simulink model "LiepkePlane"  (R2021a)
settings: Solver=FixedStepDiscrete  StartTime=0.0  StopTime=100  RelTol=1e-3  EnableMultiTasking=on
InitFcn:
  | runStart
StopFcn:
  | createGraphs
values from neighbouring files (symbols this model uses):
  alpha_matrix = data.alpha    [DatcomImport.m]
  alphai = trimAngle    (= -0.08927272)    [runStart.m]
  alt_matrix = data.alt    [DatcomImport.m]
  b = 8.0162    [runStart.m]
  beta = 0    [runStart.m]
  cbar = 4.3    [runStart.m]
  CD_0 = 0.0205    [runStart.m]
  CD_alpha = 0.058388    [runStart.m]
  CD_de = 0    [runStart.m]
  CD_ih = 0    [runStart.m]
  CD_q = 0    [runStart.m]
  CL_0 = 0.149    [runStart.m]
  Cl_0 = 0    [runStart.m]
  CL_alpha = 5.1265    [runStart.m]
  Cl_beta = -0.0301    [runStart.m]
  Cl_da = -0.1    [runStart.m]
  CL_de = 0.38    [runStart.m]
  Cl_dr = 0.05    [runStart.m]
  CL_ih = 0    [runStart.m]
  Cl_p = -0.5    [runStart.m]
  CL_q = 10.0    (= 10)    [runStart.m]
  Cl_r = 0.28    [runStart.m]
  cla_matrix = data.cla    [DatcomImport.m]
  clb_matrix = data.clb    [DatcomImport.m]
  clp_matrix = data.clp    [DatcomImport.m]
  clq_matrix = data.clq    [DatcomImport.m]
  clr_matrix = data.clr    [DatcomImport.m]
  Cm_0 = -0.08    [runStart.m]
  Cm_alpha = -0.3109    [runStart.m]
  Cm_de = -0.88    [runStart.m]
  Cm_ih = 0    [runStart.m]
  Cm_q = -17.7    [runStart.m]
  cma_matrix = data.cma    [DatcomImport.m]
  cmq_matrix = data.cmq    [DatcomImport.m]
  Cn_0 = 0    [runStart.m]
  Cn_beta = 0.1297    [runStart.m]
  Cn_da = 0.003    [runStart.m]
  Cn_dr = -0.18436    [runStart.m]
  Cn_p = - 0.09    (= -0.09)    [runStart.m]
  Cn_r = -0.26    [runStart.m]
  cnb_matrix = data.cnb    [DatcomImport.m]
  cnp_matrix = data.cnp    [DatcomImport.m]
  cnr_matrix = data.cnr    [DatcomImport.m]
  CY_0 = 0    [runStart.m]
  CY_beta = -.0301    (= -0.0301)    [runStart.m]
  CY_da = 0    [runStart.m]
  CY_dr = 0.0280    (= 0.028)    [runStart.m]
  CY_p = -0.140    (= -0.14)    [runStart.m]
  CY_r = 0.61    [runStart.m]
  cyb_matrix = data.cyb    [DatcomImport.m]
  cyp_matrix = data.cyp    [DatcomImport.m]
  H = 1981.2    [runStart.m]
  Ix = 1084.7    [runStart.m]
  Iy = 6507.9    [runStart.m]
  Iz = 7050.3    [runStart.m]
  Jxy = 0    [runStart.m]
  Jxz = 271.16    [runStart.m]
  Jyz = 0    [runStart.m]
  m = 2267.9    [runStart.m]
  mach_matrix = data.mach    [DatcomImport.m]
  p = 0    [runStart.m]
  phi = 0    [runStart.m]
  psi = 0    [runStart.m]
  q = 0    [runStart.m]
  r = 0    [runStart.m]
  S = 12.6348    [runStart.m]
  theta = trimAngle    (= -0.08927272)    [runStart.m]
  trimAngle = -8.927272e-02    (= -0.08927272)    [runStart.m]
  trimThrotte = 3.827652e-01    (= 0.3827652)    [runStart.m]
  v = 180    [runStart.m]
  xe = 0    [runStart.m]
  ye = 0    [runStart.m]
undefined symbols (not defined in the file or in its folder): DiscIntNeverNeededParam
libraries: airlib x2, aerolibfltsims x2, aerolibanimutils x2
(part 1 of 2)
settings Model: Creator=MONCAYOH  LastModifiedBy=matt
settings SolverCC: AlgebraicLoopSolver=TrustRegion
settings DataIOCC: SaveFormat=Array  SignalLoggingSaveFormat=ModelDataLogs  SaveOutput=off  SaveTime=off  ReturnWorkspaceOutputs=off
settings OptimizationCC: BlockReduction=off  BooleanDataType=off
settings DebuggingCC: SaveWithParameterizedLinksMsg=none  UnderspecifiedInitializationDetection=Classic  MergeDetectMultiDrivingBlocksExec=none  SignalResolutionControl=TryResolveAllWithWarning  MultiTaskDSMMsg=warning  MultiTaskCondExecSysMsg=none  SFMachineParentedDataDiag=warning  ArithmeticOperatorsInVariantConditions=warning
settings HardwareCC: TargetUnknown=on
settings ModelReferenceCC: PropagateSignalLabelsOutOfModel=off
settings SFSimCC: SimUseLocalCustomCode=off  CustomCodeUndefinedFunction=UseInterfaceOnly
settings RTWCC: RTWUseLocalCustomCode=off
settings CodeAppCC: StateflowObjectComments=on
settings GRTTargetCC: TargetLangStandard=C89/C90 (ANSI)  CombineOutputUpdateFcns=off  GRTInterface=on

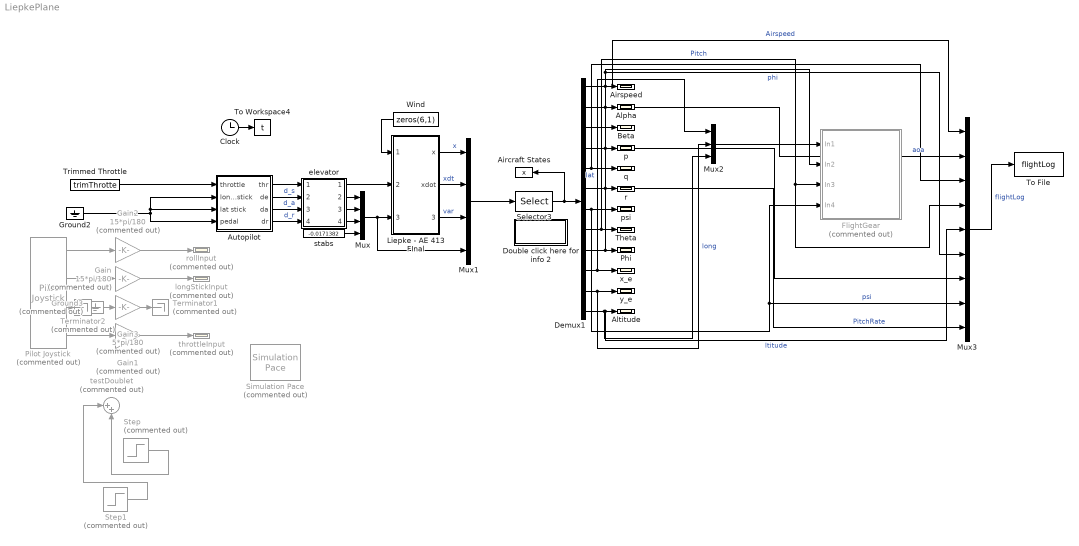
== system LiepkePlane ==
  " Liepke - AE 413 FInal" : Subsystem  AncestorBlock=airlib/B747  mask(General Nonlinear Aircraft Model){GM1=[cbar   b   S   Ix  Iy  Iz   Jxy Jxz  Jyz   m], CD_wind=[CD_0   CD_alpha   CD_q   CD_de   CD_ih], CL_wind=[CL_0   CL_alpha   CL_q   CL_de   CL_ih], Cm_body=[Cm_0   Cm_alpha   Cm_q   Cm_de   Cm_ih], CY_body=[CY_0   CY_beta   CY_p   CY_r   CY_da   CY_dr], Cl_body=[Cl_0   Cl_beta   Cl_p   Cl_r   Cl_da   Cl_dr], Cn_body=[Cn_0   Cn_beta   Cn_p   Cn_r   Cn_da   Cn_dr], x0=[v alphai beta p q r psi theta phi xe ye H]}
      mask prompts: GM1 "Geometry and Mass : [cbar   b    S    Ix   Iy   Iz   Jxy  Jxz  Jyz  m]"; CD_wind "Aerodynamic D-Force Derivatives : [CD0 CDa CDq CDde CDih]"; CL_wind "Aerodynamic L-Force Derivatives : [CL0 CLa CLq CLde CLih]"; Cm_body "Aerodynamic Y-Moment Derivatives : [Cm0 Cma Cmq Cmde Cmih]"; CY_body "Aerodynamic Y-Force Derivatives : [CY0 CYb CYp CYr CYda CYdr]"; Cl_body "Aerodynamic X-moment Derivatives : [Cl0 Clb Clp Clr Clda Cldr]"; Cn_body "Aerodynamic Z-moment Derivatives : [Cn0 Cnb Cnp Cnr Cnda Cndr]"; x0 "Initial Condition x0 [v alpha beta p q r psi theta phi xe ye H]"
      mask help:
      | The first input contains the wind velocity and acceleration.
      |   The second input contains external forces and moments in body axis.
      |   The third input contains the deflections of elevators, ailerons, rudder,
      |   and flaps. For a list of outputs look under the mask.
      |   NB : The International measurement system (MKS) is adopted.
      mask init:
      | AM=zeros(6,19);
      | AM(1,[1 2 9 11 12])=reshape(CD_wind,1,5);
      | AM(3,[1 2 9 11 12])=reshape(CL_wind,1,5);
      | AM(5,[1 2 9 11 12])=reshape(Cm_body,1,5);
      | AM(2,[1 5 8 10 13 14])=reshape(CY_body,1,6);
      | AM(4,[1 5 8 10 13 14])=reshape(Cl_body,1,6);
      | AM(6,[1 5 8 10 13 14])=reshape(Cn_body,1,6);
      | 
      | Ix=GM1(4);Iy=GM1(5);Iz=GM1(6);
      | Jxy=GM1(7);Jxz=GM1(8);Jyz=GM1(9);
      | 
      | detI = Ix*Iy*Iz - 2*Jxy*Jxz*Jyz - Ix*Jyz^2 - Iy*Jxz^2 - Iz*Jxy^2;
      | I1   = Iy*Iz - Jyz^2;I2   = Jxy*Iz + Jyz*Jxz;
      | I3   = Jxy*Jyz + Iy*Jxz;I4   = Ix*Iz - Jxz^2;
      | I5   = Ix*Jyz + Jxy*Jxz;I6   = Ix*Iy - Jxy^2;
      | 
      | Pl  = I1/detI; Pm = I2/detI; Pn = I3/detI;
      | Ppp = -(Jxz*I2 - Jxy*I3)/detI;Ppq = (Jxz*I1 - Jyz*I2 - (Iy-Ix)*I3)/detI;
      | Ppr = -(Jxy*I1 + (Ix-Iz)*I2 - Jyz*I3)/detI;Pqq = (Jyz*I1 - Jxy*I3)/detI;
      | Pqr = -((Iz-Iy)*I1 - Jxy*I2 + Jxz*I3)/detI;Prr = -(Jyz*I1 - Jxz*I2)/detI;
      | 
      | Ql  = I2/detI; Qm = I4/detI; Qn = I5/detI;
      | Qpp = -(Jxz*I4 - Jxy*I5)/detI;Qpq = (Jxz*I2 - Jyz*I4 - (Iy-Ix)*I5)/detI;
      | Qpr = -(Jxy*I2 + (Ix-Iz)*I4 - Jyz*I5)/detI;Qqq = (Jyz*I2 - Jxy*I5)/detI;
      | Qqr = -((Iz-Iy)*I2 - Jxy*I4 + Jxz*I5)/detI;Qrr = -(Jyz*I2 - Jxz*I4)/detI;
      | 
      | Rl  = I3/detI; Rm = I5/detI; Rn = I6/detI;
      | Rpp = -(Jxz*I5 - Jxy*I6)/detI;
      | Rpq = (Jxz*I3 - Jyz*I5 - (Iy-Ix)*I6)/detI;
      | Rpr = -(Jxy*I3 + (Ix-Iz)*I5 - Jyz*I6)/detI;
      | Rqq = (Jyz*I3 - Jxy*I6)/detI;
      | Rqr = -((Iz-Iy)*I3 - Jxy*I5 + Jxz*I6)/detI;
      | Rrr = -(Jyz*I3 - Jxz*I5)/detI;
      | 
      | GM2 = [  Pl   Pm   Pn   Ppp  Ppq  Ppr  Pqq  Pqr  Prr ;
      |                Ql  Qm   Qn   Qpp  Qpq  Qpr  Qqq  Qqr  Qrr ;
      |                Rl  Rm   Rn   Rpp  Rpq  Rpr  Rqq  Rqr  Rrr ];
      | 
      | xfix=1;
      mask Help:
      | <p>
      | This block is a general nonlinear 6DOF aircraft model, with a very accurate built-in atmosphere model and constant aerodynamic derivatives.
      | The architecture of the block is largely based on the Aircraft block provided by the <A
      | HREF="http://www.mathworks.com/matlabcentral/fileexchange/loadFile.do?objectId=252&objectType=file">FDC toolbox</A> (Marc Rauw, 1993-2000).
      | </p>
      | <p>
      | The geometric and inertal data of the aircraft are entered as parameters in the first row of the mask. The other six rows contains the
      | non-dimensional aerodynamic derivatives. The last row is the initial state.
      | </p>
      | <p>
      | The first input contains the wind velocity and acceleration.
      | The second input contains external forces and moments in the aircraft body axis.
      | The third input contains the deflections of elevators, ailerons, rudder,
      | and flaps or stabilators. For a list of outputs look under the mask.
      | </p>
      | <p>
      | The control surface sign conventions are the same adopted in books such as Stevens-Lewis and Etkin, and in many flight simulators,
      | including the FDC toolbox. <br>
      | Specifically, positive elevator deflection causes negative pitching moment (Cmde &#60 0), positive rudder deflection causes negative yawing
      | moment (Cndr &#60 0), and positive aileron deflection causes negative rolling moment (Clda &#60 0). Another way to say the same thing is
      | that, the positive elevators deflection is Trailing Edge Down (TED), the positive rudder(s) deflection is Trailing Edge Left (TEL), and,
      | taking as TED the positive ailerons deflection, da=K*(da_right-da_left), with K usually equal to 1 (FDC) or 1/2.
      | </p>
      | <p>
      | Since this block is largely based on the FDC toolbox, i redirect you to the FDC Toolbox manual, for a good explanation of the underlying
      | components. Besides the mask and the fact that the aerodynamic derivatives are expressed in the stability axis, the only relevant difference
      | with the FDC toolbox is that in the computation of the aerodynamic forces, q is normalized as q*cbar/2V instead of q*cbar/V. The majority
      | of aeronautics books that i've seen use q*cbar/2V.
      | </p>
      | <p>
      | Please note that the International Measurement System is adopted. So, lengths are in meters, masses in Kg, and inertia moments in Kg*m^2.
      | Moreover, forces are in N, moments in N*m, accelerations in g, and angles in radians. For those that use the english system, here are some useful
      | conversion factors: <br>
      | 1 ft   = 0.3048 m, 1 lb   = 0.4536 Kg, 1 slug = 14.593903 Kg ,  1 slug*ft^2 = 1.355818 Kg*m^2
      | <br>
      | </p>
      | <p>
      | Finally, there is an <A HREF="http://www.aae.uiuc.edu/m-selig/apasim/Aircraft-uiuc.html">excellent source</A> of aircraft aerodynamic data
      | which is mantained by Michael S. Selig, Rob Deters, and Glen Dimock at the university of Urbana-Champaign. To use any of the given models
      | you just need to type the supplied aircraft data in the block mask.
      | </p>
      | <p>
      | <p>
      | December 2002, Giampiero Campa
      | </p>
      | </p>
      mask Display: disp('General\nAircraft\nModel')
  Aircraft States : ToWorkspace  VariableName=x  SampleTime=0.05
  Airspeed : Scope
  Alpha : Scope
  Altitude : Scope
  Autopilot : Subsystem
  Beta : Scope
  Clock : Clock
  Demux1 : Demux  Outputs=12
      settings: DisplayOption=none
  Double click here for info 2 : Subsystem
      mask Display: disp('Output\nSignals')
  FlightGear : Subsystem  Commented=on
  Gain : Gain  Commented=on  Gain=15*pi/180
  Gain1 : Gain  Commented=on
  Gain2 : Gain  Commented=on  Gain=15*pi/180
  Gain3 : Gain  Commented=on  Gain=5*pi/180
  Ground2 : Ground
  Ground3 : Ground  Commented=on
  Mux : Mux
  Mux1 : Mux  Inputs=[12 12 12 4]
  Mux2 : Mux  Inputs=3
  Mux3 : Mux  Inputs=9
  Phi : Scope
  Pilot Joystick : aerolibanimutils/Pilot Joystick  Commented=on  JoystickID=Joystick1  OutputConfiguration=FourAxis  SampleTime=.05
  Selector3 : Selector  InputPortWidth=40  IndexOptions=Index vector (dialog)  Indices=1:12  OutputSizes=1
  Simulation Pace : aerolibanimutils/Simulation Pace  Commented=on  SimulationPace=1  SleepMode=Auto  OutputPaceError=off  SampleTime=-1
  Step : Step  Commented=on  Time=2  Before=-1  SampleTime=0
  Step1 : Step  Commented=on  Time=4  After=-1  SampleTime=0
  Terminator1 : Terminator  Commented=on
  Terminator2 : Terminator  Commented=on
  Theta : Scope
  To File : ToFile  Filename=flightLog  MatrixName=data  SaveFormat=Timeseries
  To Workspace4 : ToWorkspace  VariableName=t  SampleTime=-1
  Trimmed Throttle : Constant  Value=trimThrotte
  Wind : Constant  Value=zeros(6,1)
  elevator : Subsystem
      mask Display: disp('Cable &\nactuator\ndynamics')
  longStickInput : Scope  Commented=on
  p : Scope
  psi : Scope
  q : Scope
  r : Scope
  rollInput : Scope  Commented=on
  stabs : Constant  Value=-0.0171382
  testDoublet : Sum  Commented=on  Inputs=|++
  throttleInput : Scope  Commented=on
  x_e : Scope
  y_e : Scope
  wires:
  elevator/3(deltaa) -> Mux/2
  elevator/4(deltar) -> Mux/3
  elevator/2(deltae) -> Mux/1
  Autopilot/2(de) -> elevator/2(D_elv)  "d_s"
  Autopilot/3(da) -> elevator/3(D_ail)  "d_a"
  Autopilot/4(dr) -> elevator/4(D_rud)  "d_r"
  Mux/1 -> " Liepke - AE 413 FInal"/3(deflect), Mux1/4
  elevator/1(throttle) -> " Liepke - AE 413 FInal"/2(ext fm)
  Selector3/1 -> Demux1/1, Aircraft States/1
  Demux1/3 -> Beta/1
  Demux1/4 -> Mux3/7, p/1
  Demux1/5 -> q/1, Mux3/3
  Demux1/7 -> Mux3/8, FlightGear/4(In4), psi/1  "psi"
  Demux1/9 -> Mux3/6, FlightGear/2(In2), Phi/1  "phi"
  Demux1/10 -> Mux2/1, x_e/1  "lat"
  Demux1/11 -> Mux2/2, y_e/1  "long"
  Autopilot/1(thr) -> elevator/1(D_thr)
  Clock/1 -> To Workspace4/1
  stabs/1 -> Mux/4
  Wind/1 -> " Liepke - AE 413 FInal"/1(" uwind")
  " Liepke - AE 413 FInal"/1(x) -> Mux1/1  "x"
  " Liepke - AE 413 FInal"/2(xdot) -> Mux1/2  "xdt"
  " Liepke - AE 413 FInal"/3(others) -> Mux1/3  "var"
  Mux2/1 -> FlightGear/1(In1)
  Mux1/1 -> Selector3/1
  Demux1/12 -> Mux3/5, Altitude/1, Mux2/3  "ltitude"
  Demux1/2 -> Mux3/2, Alpha/1  "aoa"
  Demux1/8 -> Mux3/4, FlightGear/3(In3), Theta/1  "Pitch"
  Demux1/1 -> Mux3/1, Airspeed/1  "Airspeed"
  Mux3/1 -> To File/1  "flightLog"
  Demux1/6 -> Mux3/9, r/1  "PitchRate"
  Gain1/1 -> throttleInput/1
  Pilot Joystick/3 -> Terminator2/1
  Step1/1 -> testDoublet/1
  Step/1 -> testDoublet/2
  Gain2/1 -> rollInput/1
  Gain/1 -> longStickInput/1
  Pilot Joystick/1 -> Gain2/1
  Pilot Joystick/2 -> Gain/1
  Pilot Joystick/4 -> Gain1/1
  Ground2/1 -> Autopilot/3(lat stick), Autopilot/2(long stick), Autopilot/4(pedal)
  Trimmed Throttle/1 -> Autopilot/1(throttle)
  Gain3/1 -> Terminator1/1
  Ground3/1 -> Gain3/1

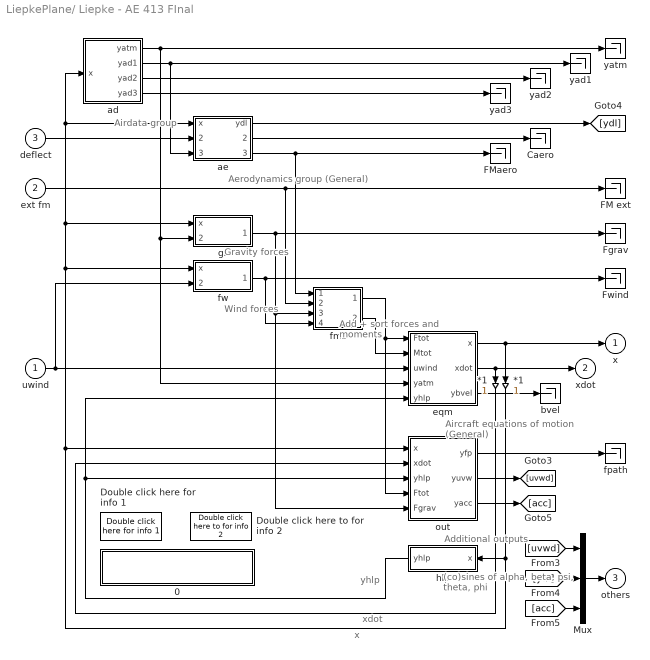
== system LiepkePlane/ Liepke - AE 413 FInal ==
  note: xdot
  note: x
  note: yhlp
  note: Additional outputs
  note: Aircraft equations
      | of motion (General)
  note: Wind forces
  note: Gravity forces
  note: Aerodynamics
      | group (General)
  note: (co)sines of
      | alpha, beta,
      | psi, theta, phi
  note: Add + sort
      | forces and
      | moments
  note: Airdata group
  " uwind" : Inport
  ext fm : Inport  Port=2
  deflect : Inport  Port=3
  " *1" : Gain  SaturateOnIntegerOverflow=on  OutDataTypeStr=Inherit: Same as input  ParamDataTypeStr=Inherit: Same as input
  *1 : Gain  SaturateOnIntegerOverflow=on  OutDataTypeStr=Inherit: Same as input  ParamDataTypeStr=Inherit: Same as input
  0 : Subsystem
      mask Display: disp('AIRCRAFT, main level\nM.O. Rauw')
  Caero : Terminator
  Double click here for info 1 : airlib/DT-B747/Double click here for info 1  SystemSampleTime=-1  VariantActivationTime=update diagram  Latency=0  AutoFrameSizeCalculation=off
  Double click here to for info 2 : airlib/DT-B747/Double click here to for info 2  SystemSampleTime=-1  VariantActivationTime=update diagram  Latency=0  AutoFrameSizeCalculation=off
  FM ext : Terminator
  FMaero : Terminator
  Fgrav : Terminator
  Fwind : Terminator
  Mux : Mux  Inputs=[3 3 6]
  ad : Subsystem
  ae : Subsystem
  bvel : Terminator
  eqm : Subsystem
  fms : Subsystem  mask(FMsort){}
      mask help: Forces and Moments sorting block
      mask Display: disp('FMsort')
  fpath : Terminator
  fw : Subsystem  mask(fwind){m=GM1(10)}
      mask prompts: m "Mass of the aircraft [kg]:"
      mask help: Forces due to non-steady atmosphere.
      mask Display: disp('Fwind')
  gr : Subsystem  mask(Gravity){m=GM1(10)}
      mask prompts: m "Mass of the aircraft [kg]:"
      mask help: Gravity forces.
      mask Display: disp('Gravity')
  hlp : Subsystem  mask(Hlpfcn){}
      mask help: Help sines and cosines
      mask Display: disp('hlpfcn')
  out : Subsystem
  yad1 : Terminator
  yad2 : Terminator
  yad3 : Terminator
  yatm : Terminator
  x : Outport
  xdot : Outport  Port=2
  others : Outport  Port=3
  wires:
  fms/1(Ftot) -> out/4(Ftot), eqm/1(Ftot)
  ext fm/1 -> fms/2(FMprop), FM ext/1
  deflect/1 -> ae/2(uaero)
  ad/4(yad3) -> yad3/1
  ae/1(ydl) -> [ydl]
  ae/2(Caero) -> Caero/1
  eqm/3(ybvel) -> bvel/1
  out/1(yfp) -> fpath/1
  ad/2(yad1) -> ae/3(yad1), yad1/1
  ad/3(yad2) -> yad2/1
  ad/1(yatm) -> eqm/4(yatm), gr/2(yatm), yatm/1
  out/3(yacc) -> [acc]
  fw/1(Fwind) -> Fwind/1, fms/4(Fwind)
  ae/3(FMaero) -> FMaero/1, fms/1(FMaero)
  hlp/1(yhlp) -> eqm/5(yhlp), out/3(yhlp)
  " uwind"/1 -> eqm/3(uwind), fw/2(uwind)
  *1/1 -> out/2(xdot)
  gr/1(Fgrav) -> fms/3(Fgrav), out/5(Fgrav), Fgrav/1
  " *1"/1 -> hlp/1(x), out/1(x), fw/1(x), gr/1(x), ae/1(x), ad/1(x)
  eqm/2(xdot) -> xdot/1, *1/1
  eqm/1(x) -> x/1, " *1"/1
  fms/2(Mtot) -> eqm/2(Mtot)
  out/2(yuvw) -> [uvwd]
  [uvwd] -> Mux/1
  [ydl] -> Mux/2
  [acc] -> Mux/3
  Mux/1 -> others/1

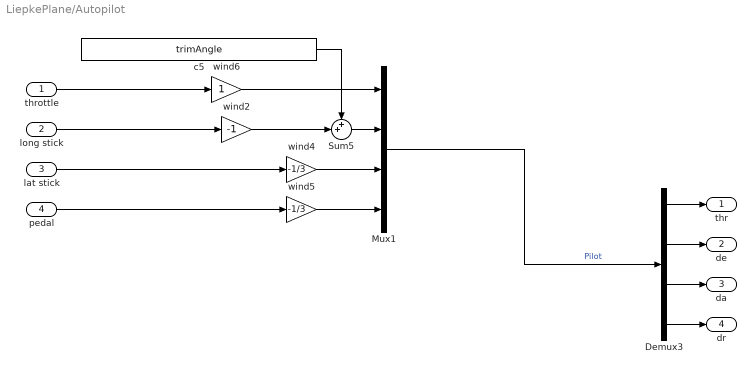
== system LiepkePlane/Autopilot ==
  throttle : Inport
  long stick : Inport  Port=2
  lat stick : Inport  Port=3
  pedal : Inport  Port=4
  Demux3 : Demux
      settings: DisplayOption=none
  Mux1 : Mux
  Sum5 : Sum  Inputs=++|  InputSameDT=on  SaturateOnIntegerOverflow=on  OutDataTypeStr=Inherit: Same as first input
  c5 : Constant  Value=trimAngle
  wind2 : Gain  Gain=-1  SaturateOnIntegerOverflow=on  OutDataTypeStr=Inherit: Same as input  ParamDataTypeStr=Inherit: Same as input
  wind4 : Gain  Gain=-1/3  SaturateOnIntegerOverflow=on  OutDataTypeStr=Inherit: Same as input  ParamDataTypeStr=Inherit: Same as input
  wind5 : Gain  Gain=-1/3  SaturateOnIntegerOverflow=on  OutDataTypeStr=Inherit: Same as input  ParamDataTypeStr=Inherit: Same as input
  wind6 : Gain  SaturateOnIntegerOverflow=on  OutDataTypeStr=Inherit: Same as input  ParamDataTypeStr=Inherit: Same as input
  thr : Outport  VectorParamsAs1DForOutWhenUnconnected=off
  de : Outport  Port=2  VectorParamsAs1DForOutWhenUnconnected=off
  da : Outport  Port=3  VectorParamsAs1DForOutWhenUnconnected=off
  dr : Outport  Port=4  VectorParamsAs1DForOutWhenUnconnected=off
  wires:
  long stick/1 -> wind2/1
  lat stick/1 -> wind4/1
  pedal/1 -> wind5/1
  Mux1/1 -> Demux3/1  "Pilot"
  Demux3/1 -> thr/1
  Demux3/2 -> de/1
  Demux3/3 -> da/1
  Demux3/4 -> dr/1
  wind4/1 -> Mux1/3
  wind5/1 -> Mux1/4
  throttle/1 -> wind6/1
  c5/1 -> Sum5/1
  Sum5/1 -> Mux1/2
  wind2/1 -> Sum5/2
  wind6/1 -> Mux1/1

== system LiepkePlane/Double click here for info 2 ==
  note: 01 v (m/s)
      | 02 alpha (rad)
      | 03 beta (rad)
      | 04 p (rad/s)
      | 05 q (rad/s)
      | 06 r  (rad/s)
      | 07 psi (rad)
      | 08 theta (rad)
      | 09 phi (rad)
      | 10 xe (m)
      | 11 ye (m)
      | 12 ze (m)
      | 13 v dot (m/s2)
      | 14 alpha dot (rad/s)
      | 15 beta dot (rad/s)
      | 16 p dot (rad/s2)
      | 17 q dot (rad/s2)
      | 18 r dot (rad/s2)
      | 19 fi dot (rad/s)
      | 20 theta dot (rad/s)
      | 21 psi dot (rad/s)
      | 22 xe dot (m/s)
      | 23 ye dot (m/s)
      | 24 ze dot (m/s)
      | 25 u dot (m/s2)
      | 26 v dot (m/s2)
      | 27 w dot (m/s2)
      | 28 pb/2v (rad)
      | 29 qc/v (rad)
      | 30 rb/v (rad)
      | 31 Ax (g)
      | 32 Ay (g)
      | 33 Az (g)
      | 34 ax (g)
      | 35 ay (g)
      | 36 az (g)
      | 37 delta elevators (rad)
      | 38 delta ailerons (rad)
      | 39 delta rudder (rad)
      | 40 delta stabs (rad)

== system LiepkePlane/FlightGear ==
  In1 : Inport
  In2 : Inport  Port=2
  In3 : Inport  Port=3
  In4 : Inport  Port=4
  Data Type Conversion : DataTypeConversion  OutDataTypeStr=single
  Data Type Conversion1 : DataTypeConversion  OutDataTypeStr=single
  Data Type Conversion2 : DataTypeConversion  OutDataTypeStr=single
  Lat,Lon,Elev Convertor : Subsystem
  Pack net_fdm Packet for FlightGear : aerolibfltsims/Pack net_fdm Packet for FlightGear  FlightGearVersion=v2.4  ShowPositionAttitudeInputs=on  ShowVelocityAccelerationInputs=off  ShowControlSurfacePositionInputs=off  ShowEngineFuelInputs=off  ShowLandingGearInputs=off  ShowEnvironmentInputs=off  SampleTime=-1  packetVersion=24
      settings: SourceProductBaseCode=AE
  Send net_fdm Packet to FlightGear : aerolibfltsims/Send net_fdm Packet to FlightGear  DestinationIpAddress=127.0.0.1  DestinationPort=5502  LocalIpPort=-1  varLen=off  SampleTime=-1
      settings: SourceProductBaseCode=AE
  wires:
  In2/1 -> Data Type Conversion2/1
  In3/1 -> Data Type Conversion1/1
  Lat,Lon,Elev Convertor/2(Lat) -> Pack net_fdm Packet for FlightGear/2
  Lat,Lon,Elev Convertor/3(Ele) -> Pack net_fdm Packet for FlightGear/3
  In1/1 -> Lat,Lon,Elev Convertor/1(Inp)
  Data Type Conversion1/1 -> Pack net_fdm Packet for FlightGear/5
  Data Type Conversion2/1 -> Pack net_fdm Packet for FlightGear/4
  Lat,Lon,Elev Convertor/1(Lon) -> Pack net_fdm Packet for FlightGear/1
  In4/1 -> Data Type Conversion/1
  Data Type Conversion/1 -> Pack net_fdm Packet for FlightGear/6
  Pack net_fdm Packet for FlightGear/1 -> Send net_fdm Packet to FlightGear/1

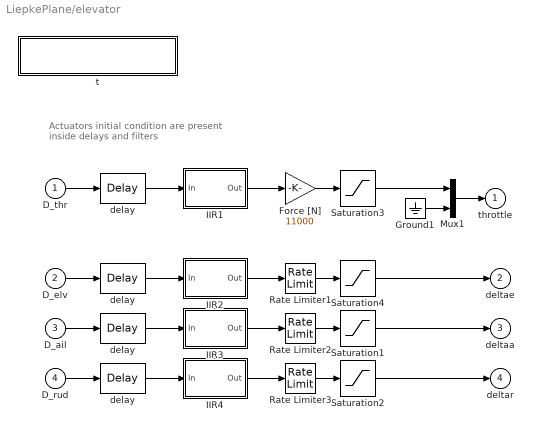
== system LiepkePlane/elevator ==
  note: Actuators initial condition are present
      | inside delays and filters
  D_thr : Inport
  D_elv : Inport  Port=2
  D_ail : Inport  Port=3
  D_rud : Inport  Port=4
  " delay" : TransportDelay  DelayTime=0.03  InitialOutput=-1.71374e-004
  " delay " : TransportDelay  DelayTime=0.03  InitialOutput=0.490154
  Force [N] : Gain  Gain=11000  SaturateOnIntegerOverflow=on  OutDataTypeStr=Inherit: Same as input  ParamDataTypeStr=Inherit: Same as input
  Ground1 : Ground
  IIR1 : Subsystem  mask(Discrete Time First Order IIR){ni=1, a=4, x0=0.490154, T=0.05}
      mask prompts: ni "Number of Channels"; a "Cutoff Frequency (a)"; x0 "Initial Condition"; T "Sample Time"
      mask help:
      | Each channel has the transfer function
      |   (1-exp(-aT))/(1-exp(-aT)(z^-1)) which is a good
      |   (pz-matched) approximation of a/(s+a) if 10*a*T<pi
      mask init:
      | A=[];B=[];C=[];D=[];
      | for i=1:ni,
      | A=[A,zeros(size(A,1),1);zeros(1,size(A,2)),exp(-a*T)];
      | B=[B,zeros(size(B,1),1);zeros(1,size(B,2)),1-exp(-a*T)];
      | C=[C,zeros(size(C,1),1);zeros(1,size(C,2)),exp(-a*T)];
      | D=[D,zeros(size(D,1),1);zeros(1,size(D,2)),1-exp(-a*T)];
      | end
      mask Help:
      | <p>
      |   Each channel has the transfer function
      |   (1-exp(-aT))/(1-exp(-aT)(z^-1)) which is a good
      |   (pz-matched) approximation of a/(s+a) if 10*a*T<pi
      | </p>
      mask Display: dpoly(a,[1 a],'s')
  IIR2 : Subsystem  mask(Discrete Time First Order IIR){ni=1, a=15, x0=-1.71374e-004, T=0.05}
      mask prompts: ni "Number of Channels"; a "Cutoff Frequency (a)"; x0 "Initial Condition"; T "Sample Time"
      mask help:
      | Each channel has the transfer function
      |   (1-exp(-aT))/(1-exp(-aT)(z^-1)) which is a good
      |   (pz-matched) approximation of a/(s+a) if 10*a*T<pi
      mask init: same as LiepkePlane/elevator/IIR1
      mask Help:
      | <p>
      |   Each channel has the transfer function
      |   (1-exp(-aT))/(1-exp(-aT)(z^-1)) which is a good
      |   (pz-matched) approximation of a/(s+a) if 10*a*T<pi
      | </p>
      mask Display: dpoly(a,[1 a],'s')
  IIR3 : Subsystem  mask(Discrete Time First Order IIR){ni=1, a=40, x0=0, T=0.05}
      mask prompts: ni "Number of Channels"; a "Cutoff Frequency (a)"; x0 "Initial Condition"; T "Sample Time"
      mask help:
      | Each channel has the transfer function
      |   (1-exp(-aT))/(1-exp(-aT)(z^-1)) which is a good
      |   (pz-matched) approximation of a/(s+a) if 10*a*T<pi
      mask init: same as LiepkePlane/elevator/IIR1
      mask Help:
      | <p>
      |   Each channel has the transfer function
      |   (1-exp(-aT))/(1-exp(-aT)(z^-1)) which is a good
      |   (pz-matched) approximation of a/(s+a) if 10*a*T<pi
      | </p>
      mask Display: dpoly(a,[1 a],'s')
  IIR4 : Subsystem  mask(Discrete Time First Order IIR){ni=1, a=15, x0=0, T=0.05}
      mask prompts: ni "Number of Channels"; a "Cutoff Frequency (a)"; x0 "Initial Condition"; T "Sample Time"
      mask help:
      | Each channel has the transfer function
      |   (1-exp(-aT))/(1-exp(-aT)(z^-1)) which is a good
      |   (pz-matched) approximation of a/(s+a) if 10*a*T<pi
      mask init: same as LiepkePlane/elevator/IIR1
      mask Help:
      | <p>
      |   Each channel has the transfer function
      |   (1-exp(-aT))/(1-exp(-aT)(z^-1)) which is a good
      |   (pz-matched) approximation of a/(s+a) if 10*a*T<pi
      | </p>
      mask Display: dpoly(a,[1 a],'s')
  Mux1 : Mux  Inputs=[1 5]
  Rate Limiter1 : RateLimiter  RisingSlewLimit=100*pi/180  FallingSlewLimit=-100*pi/180
  Rate Limiter2 : RateLimiter  RisingSlewLimit=100*pi/180  FallingSlewLimit=-100*pi/180
  Rate Limiter3 : RateLimiter  RisingSlewLimit=100*pi/180  FallingSlewLimit=-100*pi/180
  Saturation1 : Saturate  UpperLimit=20*pi/180  LowerLimit=-20*pi/180
  Saturation2 : Saturate  UpperLimit=20*pi/180  LowerLimit=-20*pi/180
  Saturation3 : Saturate  UpperLimit=245440  LowerLimit=0
  Saturation4 : Saturate  UpperLimit=20*pi/180  LowerLimit=-20*pi/180
  delay : TransportDelay  DelayTime=0.03
  "delay " : TransportDelay  DelayTime=0.03
  t : Subsystem
      settings: OpenFcn=fdchelp actuatr
      mask Display: disp('Actuator & cable dynamics\nMarc Rauw, October 1997')
  throttle : Outport  VectorParamsAs1DForOutWhenUnconnected=off
  deltae : Outport  Port=2  VectorParamsAs1DForOutWhenUnconnected=off
  deltaa : Outport  Port=3  VectorParamsAs1DForOutWhenUnconnected=off
  deltar : Outport  Port=4  VectorParamsAs1DForOutWhenUnconnected=off
  wires:
  D_ail/1 -> delay/1
  D_elv/1 -> " delay"/1
  D_rud/1 -> "delay "/1
  IIR2/1(Out) -> Rate Limiter1/1
  Saturation4/1 -> deltae/1
  IIR3/1(Out) -> Rate Limiter2/1
  Saturation1/1 -> deltaa/1
  IIR4/1(Out) -> Rate Limiter3/1
  Saturation2/1 -> deltar/1
  Rate Limiter1/1 -> Saturation4/1
  Rate Limiter2/1 -> Saturation1/1
  Rate Limiter3/1 -> Saturation2/1
  Mux1/1 -> throttle/1
  Saturation3/1 -> Mux1/1
  Ground1/1 -> Mux1/2
  D_thr/1 -> " delay "/1
  IIR1/1(Out) -> Force [N]/1
  Force [N]/1 -> Saturation3/1
  " delay "/1 -> IIR1/1(In)
  " delay"/1 -> IIR2/1(In)
  delay/1 -> IIR3/1(In)
  "delay "/1 -> IIR4/1(In)

== system LiepkePlane/ Liepke - AE 413 FInal/0 ==

== system LiepkePlane/ Liepke - AE 413 FInal/ad ==
  x : Inport
  0 : Subsystem
      mask Display: disp('AIRDATA GROUP (level 3)\nM.O. Rauw')
  ad1 : Subsystem  mask(Airdata1){}
      mask help: Basic airdata variables
      mask Display: disp('Airdata1')
  ad2 : Subsystem  mask(Airdata2){}
      mask help: More airdata variables
      mask Display: disp('Airdata2')
  ad3 : Subsystem  mask(Airdata3){cbar=GM1(1)}
      mask prompts: cbar "Mean aerodynamic chord [m]:"
      mask help: More airdata variables
      mask Display: disp('Airdata3')
  atm : Subsystem  mask(Atmosph){}
      mask help: Atmosphere variables
      mask Display: disp('Atmosph')
  yatm : Outport
  yad1 : Outport  Port=2
  yad2 : Outport  Port=3
  yad3 : Outport  Port=4
  wires:
  ad2/1(yad2) -> yad2/1
  ad3/1(yad3) -> yad3/1
  x/1 -> atm/1(x), ad1/1(x), ad3/1(x)
  atm/1(yatm) -> yatm/1, ad1/2(yatm), ad2/1(yatm), ad3/2(yatm)
  ad1/1(yad1) -> yad1/1, ad2/2(yad1), ad3/3(yad1)

== system LiepkePlane/ Liepke - AE 413 FInal/ae ==
  x : Inport
  uaero : Inport  Port=2
  yad1 : Inport  Port=3
  0 : Subsystem
      mask Display: disp('AERODYNAMICS GROUP (level 3)\nM.O. Rauw')
  aero : Subsystem  mask(Aeromod){}
      mask help: Aerodynamic model of the DHC-2 'Beaver'.
      mask Display: disp('Aeromod\n(General)')
  dl : Subsystem  mask(Dimless){cbar=GM1(1), b=GM1(2)}
      mask prompts: cbar "Mean aerodynamic chord [m]:"; b "Wing span [m]:"
      mask help: Dimensionless rotational velocities.
      mask Display: disp('Dimless')
  fmdims : Subsystem  mask(FMdims){cbar=GM1(1), b=GM1(2), S=GM1(3)}
      mask prompts: cbar "Mean aerodynamic chord [m]:"; b "Wing span [m]:"; S "Wing surface [m^2]:"
      mask help:
      | Calculate forces and moments from
      | dimensionless derivatives.
      mask Display: disp('FMdims')
  ydl : Outport
  Caero : Outport  Port=2
  FMaero : Outport  Port=3
  wires:
  aero/1(Caero) -> Caero/1, fmdims/2(Force / moment derivatives)
  dl/1(ydl) -> aero/3(ydl), ydl/1
  x/1 -> aero/1(x), dl/1(x)
  uaero/1 -> aero/2(uaero)
  yad1/1 -> aero/4(Input), fmdims/1(yad1)
  fmdims/1(Forces and moments) -> FMaero/1

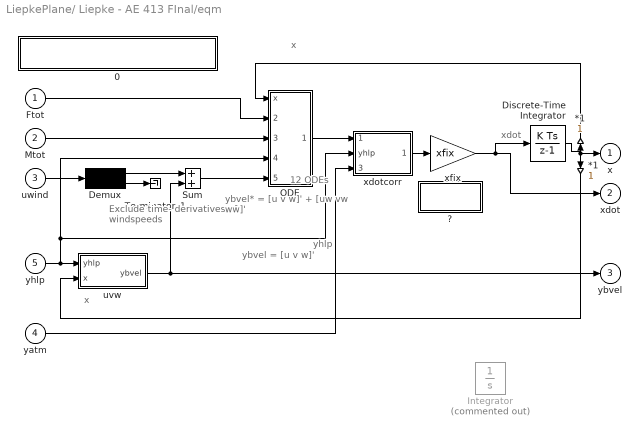
== system LiepkePlane/ Liepke - AE 413 FInal/eqm ==
  note: Exclude time-
      | derivatives
      | of windspeeds
  note: ybvel* =
      | [u v w]' +
      | [uw vw ww]'
  note: xdot
  note: x
  note: x
  note: yhlp
  note: ybvel = [u v w]'
  note: 12 ODEs
  Ftot : Inport
  Mtot : Inport  Port=2
  uwind : Inport  Port=3
  yatm : Inport  Port=4
  yhlp : Inport  Port=5
  " *1" : Gain  SaturateOnIntegerOverflow=on  OutDataTypeStr=Inherit: Same as input  ParamDataTypeStr=Inherit: Same as input
  *1 : Gain  SaturateOnIntegerOverflow=on  OutDataTypeStr=Inherit: Same as input  ParamDataTypeStr=Inherit: Same as input
  0 : Subsystem
      mask Display: disp('EQUATIONS OF MOTION (level 3)\nM.O. Rauw')
  "?" : Subsystem
      mask Display: disp('More info\nfor xfix')
  Demux : Demux  Outputs=[3 3]
      settings: DisplayOption=none
  Discrete-Time Integrator : DiscreteIntegrator  InitialCondition=x0  SampleTime=-1  ICPrevOutput=DiscIntNeverNeededParam  ICPrevScaledInput=DiscIntNeverNeededParam
  Integrator : Integrator  Commented=on  InitialCondition=x0
  ODE : Subsystem
  Sum : Sum  InputSameDT=on  SaturateOnIntegerOverflow=on  OutDataTypeStr=Inherit: Same as first input
  Terminator_1 : Terminator
  uvw : Subsystem  mask(uvw){}
      mask help:
      | Calculation of body-axes velocities
      | u, v, and w
      mask Display: disp('Body-axes\nvelocities')
  xdotcorr : Subsystem  mask(xdotcorr){b=GM1(2), S=GM1(3), m=GM1(10), CYbdot=AM(2,19)}
      mask prompts: b "Wing span [m]:"; S "Wing surface [m^2]:"; m "Mass of the aircraft [kg]:"; CYbdot "Stability-derivative CYbdot:"
      mask help:
      | Correction block to write state
      | equations for DHC-2 Beaver aircraft
      | explicitly.
      mask Display: disp('xdotcorr\n(General)')
  xfix : Gain  Gain=xfix  SaturateOnIntegerOverflow=on  OutDataTypeStr=Inherit: Same as input  ParamDataTypeStr=Inherit: Same as input
  x : Outport
  xdot : Outport  Port=2
  ybvel : Outport  Port=3
  wires:
  Demux/2 -> Terminator_1/1
  yhlp/1 -> uvw/1(yhlp), ODE/4(yhlp), xdotcorr/2(yhlp)
  ODE/1(xdot) -> xdotcorr/1(xdot uncorrected)
  Sum/1 -> ODE/5(ybvel*)
  uvw/1(ybvel) -> ybvel/1, Sum/2
  uwind/1 -> Demux/1
  Demux/1 -> Sum/1
  xdotcorr/1(xdot corrected) -> xfix/1
  yatm/1 -> xdotcorr/3(yatm)
  Ftot/1 -> ODE/2(Ftot)
  Mtot/1 -> ODE/3(Mtot)
  *1/1 -> uvw/2(x)
  Discrete-Time Integrator/1 -> x/1, " *1"/1, *1/1
  xfix/1 -> xdot/1, Discrete-Time Integrator/1
  " *1"/1 -> ODE/1(x)

== system LiepkePlane/ Liepke - AE 413 FInal/fms ==
  FMaero : Inport
  FMprop : Inport  Port=2
  Fgrav : Inport  Port=3
  Fwind : Inport  Port=4
  0 : Subsystem
      mask Display: disp('FMSORT\nM.O. Rauw, October 1997')
  Demux : Demux  Outputs=[3 3]
      settings: DisplayOption=none
  Demux1 : Demux  Outputs=[3 3]
      settings: DisplayOption=none
  Sum1 : Sum  InputSameDT=on  SaturateOnIntegerOverflow=on  OutDataTypeStr=Inherit: Same as first input
  Sum3 : Sum  Inputs=++++  InputSameDT=on  SaturateOnIntegerOverflow=on  OutDataTypeStr=Inherit: Same as first input
  Ftot : Outport
  Mtot : Outport  Port=2
  wires:
  FMaero/1 -> Demux/1
  FMprop/1 -> Demux1/1
  Demux1/2 -> Sum1/2
  Demux/2 -> Sum1/1
  Fgrav/1 -> Sum3/3
  Demux1/1 -> Sum3/2
  Sum3/1 -> Ftot/1
  Sum1/1 -> Mtot/1
  Demux/1 -> Sum3/1
  Fwind/1 -> Sum3/4

== system LiepkePlane/ Liepke - AE 413 FInal/fw ==
  x : Inport
  uwind : Inport  Port=2
  -Xw/m : Fcn  Expr=u[16] + u[5]*u[15] - u[6]*u[14]
  -Yw/m : Fcn  Expr=u[17] - u[4]*u[15] + u[6]*u[13]
  -Zw/m : Fcn  Expr=u[18] + u[4]*u[14] - u[5]*u[13]
  0 : Subsystem
      mask Display: disp('FWIND\nM.O. Rauw, Dec. 1996')
  Mux : Mux  Inputs=3
  Mux1 : Mux  Inputs=[12 6]
  gain : Gain  Gain=-m  SaturateOnIntegerOverflow=on  OutDataTypeStr=Inherit: Same as input  ParamDataTypeStr=Inherit: Same as input
  Fwind : Outport
  wires:
  uwind/1 -> Mux1/2
  x/1 -> Mux1/1
  gain/1 -> Fwind/1
  Mux/1 -> gain/1
  Mux1/1 -> -Yw/m/1, -Zw/m/1, -Xw/m/1
  -Yw/m/1 -> Mux/2
  -Xw/m/1 -> Mux/1
  -Zw/m/1 -> Mux/3

== system LiepkePlane/ Liepke - AE 413 FInal/gr ==
  x : Inport
  yatm : Inport  Port=2
  0 : Subsystem
      mask Display: disp('GRAVITY\nM.O. Rauw, October 1997')
  Mux : Mux  Inputs=3
  Mux1 : Mux  Inputs=[12 5]
  Xgr : Fcn  Expr=-m*u[17]*sin(u[8])
  Ygr : Fcn  Expr=m*u[17]*cos(u[8])*sin(u[9])
  Zgr : Fcn  Expr=m*u[17]*cos(u[8])*cos(u[9])
  Fgrav : Outport
  wires:
  Xgr/1 -> Mux/1
  Ygr/1 -> Mux/2
  Mux/1 -> Fgrav/1
  Mux1/1 -> Ygr/1, Xgr/1, Zgr/1
  Zgr/1 -> Mux/3
  x/1 -> Mux1/1
  yatm/1 -> Mux1/2

== system LiepkePlane/ Liepke - AE 413 FInal/hlp ==
  x : Inport
  0 : Subsystem
      mask Display: disp('HELP FUNCTIONS\n(often used sines and cosines)\nM.O. Rauw, October 1997')
  Mux : Mux  Inputs=11
  cos alpha : Fcn  Expr=cos(u[2])
  cos beta : Fcn  Expr=cos(u[3])
  cos phi : Fcn  Expr=cos(u[9])
  cos psi : Fcn  Expr=cos(u[7])
  cos theta : Fcn  Expr=cos(u[8])
  sin alpha : Fcn  Expr=sin(u[2])
  sin beta : Fcn  Expr=sin(u[3])
  sin phi : Fcn  Expr=sin(u[9])
  sin psi : Fcn  Expr=sin(u[7])
  sin theta : Fcn  Expr=sin(u[8])
  tan beta : Fcn  Expr=tan(u[3])
  yhlp : Outport
  wires:
  x/1 -> sin psi/1, sin beta/1, cos beta/1, sin alpha/1, cos alpha/1, tan beta/1, sin theta/1, cos theta/1, sin phi/1, cos phi/1, cos psi/1
  cos alpha/1 -> Mux/1
  sin alpha/1 -> Mux/2
  cos beta/1 -> Mux/3
  sin beta/1 -> Mux/4
  tan beta/1 -> Mux/5
  sin psi/1 -> Mux/6
  cos psi/1 -> Mux/7
  sin theta/1 -> Mux/8
  cos theta/1 -> Mux/9
  sin phi/1 -> Mux/10
  Mux/1 -> yhlp/1
  cos phi/1 -> Mux/11

== system LiepkePlane/ Liepke - AE 413 FInal/out ==
  note: Flightpath
      | variables
  note: du/dt, dv/dt, dw/dt
      | (output equations!)
  note: Body-axes accelerations
      | and specific forces
  x : Inport
  xdot : Inport  Port=2
  yhlp : Inport  Port=3
  Ftot : Inport  Port=4
  Fgrav : Inport  Port=5
  0 : Subsystem
      mask Display: disp('Additional outputs (level 3)\nM.O. Rauw')
  accel : Subsystem  mask(accel){m=GM1(10)}
      mask prompts: m "Mass of the aircraft [kg]:"
      mask help:
      | Body axes accelerations and
      | specific forces.
      mask Display: disp('Accel')
  fp : Subsystem  mask(Flpath){alpha0=x0(2)}
      mask prompts: alpha0 "Initial value of angle of attack, alpha0:"
      mask help: Flightpath related parameters.
      mask Display: disp('flpath')
  uvwdot : Subsystem  mask(uvwdot){}
      mask help: Calculation of du/dt, dv/dt, and dw/dt.
      mask Display: disp('uvwdot')
  yfp : Outport
  yuvw : Outport  Port=2
  yacc : Outport  Port=3
  wires:
  fp/1(yfp) -> yfp/1
  uvwdot/1(yuvw = [udot; vdot; wdot]) -> yuvw/1
  yhlp/1 -> uvwdot/3(yhlp)
  Ftot/1 -> accel/1(Ftot)
  accel/1(yacc) -> yacc/1
  xdot/1 -> fp/2(xdot), uvwdot/2(xdot)
  x/1 -> fp/1(x), uvwdot/1(x)
  Fgrav/1 -> accel/2(Fgrav)

== system LiepkePlane/FlightGear/Lat,Lon,Elev Convertor ==
  Inp : Inport
  Constant : Constant  Value=6380000
  Demux : Demux  Outputs=3
      settings: DisplayOption=none
  Product : Product  Inputs=/*  SaturateOnIntegerOverflow=on  OutDataTypeStr=Inherit: Same as first input
  Product1 : Product  Inputs=*//  SaturateOnIntegerOverflow=on  OutDataTypeStr=Inherit: Same as first input
  Reference Altitude : Constant  Value=0
  Reference Latitude : Constant  Value=37.7889/57.3
  Reference Longitude : Constant  Value=-122.4778/57.3
  Sum : Sum  Inputs=|++  SaturateOnIntegerOverflow=on
  Sum1 : Sum  Inputs=|++  SaturateOnIntegerOverflow=on
  Sum2 : Sum  Inputs=|++  SaturateOnIntegerOverflow=on
  Trigonometric Function : Trigonometry  Operator=cos
  Lon : Outport
  Lat : Outport  Port=2
  Ele : Outport  Port=3
  wires:
  Reference Latitude/1 -> Sum2/1
  Sum1/1 -> Lon/1
  Reference Longitude/1 -> Sum1/2
  Product1/1 -> Sum1/1
  Trigonometric Function/1 -> Product1/3
  Demux/2 -> Product1/1
  Demux/3 -> Sum/1
  Sum2/1 -> Lat/1, Trigonometric Function/1
  Product/1 -> Sum2/2
  Demux/1 -> Product/2
  Constant/1 -> Product1/2, Product/1
  Reference Altitude/1 -> Sum/2
  Sum/1 -> Ele/1
  Inp/1 -> Demux/1

== system LiepkePlane/elevator/IIR1 ==
  In : Inport
  Discrete State-Space : DiscreteStateSpace  A=A  B=B  C=C  D=D  InitialCondition=x0  SampleTime=-1
  Out : Outport  VectorParamsAs1DForOutWhenUnconnected=off
  wires:
  Discrete State-Space/1 -> Out/1
  In/1 -> Discrete State-Space/1

== system LiepkePlane/elevator/IIR2 ==
  In : Inport
  Discrete State-Space : DiscreteStateSpace  A=A  B=B  C=C  D=D  InitialCondition=x0  SampleTime=T
  Out : Outport  VectorParamsAs1DForOutWhenUnconnected=off
  wires:
  Discrete State-Space/1 -> Out/1
  In/1 -> Discrete State-Space/1

== system LiepkePlane/elevator/IIR3 ==
  In : Inport
  Discrete State-Space : DiscreteStateSpace  A=A  B=B  C=C  D=D  InitialCondition=x0  SampleTime=T
  Out : Outport  VectorParamsAs1DForOutWhenUnconnected=off
  wires:
  Discrete State-Space/1 -> Out/1
  In/1 -> Discrete State-Space/1

== system LiepkePlane/elevator/IIR4 ==
  In : Inport
  Discrete State-Space : DiscreteStateSpace  A=A  B=B  C=C  D=D  InitialCondition=x0  SampleTime=T
  Out : Outport  VectorParamsAs1DForOutWhenUnconnected=off
  wires:
  Discrete State-Space/1 -> Out/1
  In/1 -> Discrete State-Space/1

== system LiepkePlane/elevator/t ==

== system LiepkePlane/ Liepke - AE 413 FInal/ad/0 ==

== system LiepkePlane/ Liepke - AE 413 FInal/ad/ad1 ==
  x : Inport
  yatm : Inport  Port=2
  0 : Subsystem
      mask Display: disp('AIRDATA1\nM.O. Rauw, October 1997')
  M : Fcn  Expr=u[2]/u[1]
  Mux : Mux  Inputs=[1 12]
  Mux1 : Mux  Inputs=[12 5]
  Mux2 : Mux  Inputs=3
  a : Fcn  Expr=sqrt(401.8743*u[3])
  qdyn : Fcn  Expr=0.5*u[13]*u[1]^2
  yad1 : Outport
  wires:
  Mux2/1 -> yad1/1
  qdyn/1 -> Mux2/3
  a/1 -> Mux/1, Mux2/1
  M/1 -> Mux2/2
  Mux1/1 -> qdyn/1
  Mux/1 -> M/1
  x/1 -> Mux/2, Mux1/1
  yatm/1 -> a/1, Mux1/2

== system LiepkePlane/ Liepke - AE 413 FInal/ad/ad2 ==
  yatm : Inport
  yad1 : Inport  Port=2
  0 : Subsystem
      mask Display: disp('AIRDATA2\nM.O. Rauw, October 1997')
  Mux : Mux  Inputs=[5 3]
  Mux1 : Mux  Inputs=3
  Vc : Fcn  Expr=sqrt(579000*((1+u[1]/101325)^(1/3.5)-1))
  Ve : Fcn  Expr=sqrt(u[8] * 1.63265)
  qc : Fcn  Expr=u[2] * ((1+0.2*u[7]^2)^3.5-1)
  yad2 : Outport
  wires:
  yad1/1 -> Mux/2
  yatm/1 -> Mux/1
  Mux/1 -> qc/1, Ve/1
  Ve/1 -> Mux1/2
  Vc/1 -> Mux1/3
  qc/1 -> Vc/1, Mux1/1
  Mux1/1 -> yad2/1

== system LiepkePlane/ Liepke - AE 413 FInal/ad/ad3 ==
  x : Inport
  yatm : Inport  Port=2
  yad1 : Inport  Port=3
  0 : Subsystem
      mask Display: disp('AIRDATA3\nM.O. Rauw, October 1997')
  Mux : Mux  Inputs=3
  Mux1 : Mux  Inputs=[12 5 3]
  Re : Fcn  Expr=(u[13]*u[1])/u[16]
  Tt : Fcn  Expr=u[15] * (1+0.2*u[19]^2)
  cbar : Gain  Gain=cbar  SaturateOnIntegerOverflow=on  OutDataTypeStr=Inherit: Same as input  ParamDataTypeStr=Inherit: Same as input
  yad3 : Outport
  wires:
  yad1/1 -> Mux1/3
  yatm/1 -> Mux1/2
  x/1 -> Mux1/1
  Re/1 -> Mux/2, cbar/1
  Mux1/1 -> Re/1, Tt/1
  Mux/1 -> yad3/1
  Tt/1 -> Mux/1
  cbar/1 -> Mux/3

== system LiepkePlane/ Liepke - AE 413 FInal/ad/atm ==
  x : Inport
  0 : Subsystem
      mask Display: disp('ATMOSPH\nM.O. Rauw, October 1997')
  Mux : Mux  Inputs=2
  Mux1 : Mux  Inputs=[2 1]
  Mux2 : Mux  Inputs=5
  T : Fcn  Expr=288.15 - 0.0065*u[12]
  g : Fcn  Expr=9.80665*(6371020/(6371020+u[12]))^2
  mu : Fcn  Expr=(1.458*10^(-6)*u[2]^1.5)/(u[2]+110.4)
  ps : Fcn  Expr=101325*(u[2]/288.15)^(u[1]/1.86584)
  rho : Fcn  Expr=u[3]/(287.053*u[2])
  yatm : Outport
  wires:
  x/1 -> T/1, g/1
  Mux/1 -> Mux1/1, mu/1, ps/1
  ps/1 -> Mux1/2, Mux2/2
  T/1 -> Mux/2, Mux2/3
  g/1 -> Mux/1, Mux2/5
  rho/1 -> Mux2/1
  Mux1/1 -> rho/1
  Mux2/1 -> yatm/1
  mu/1 -> Mux2/4

== system LiepkePlane/ Liepke - AE 413 FInal/ae/0 ==

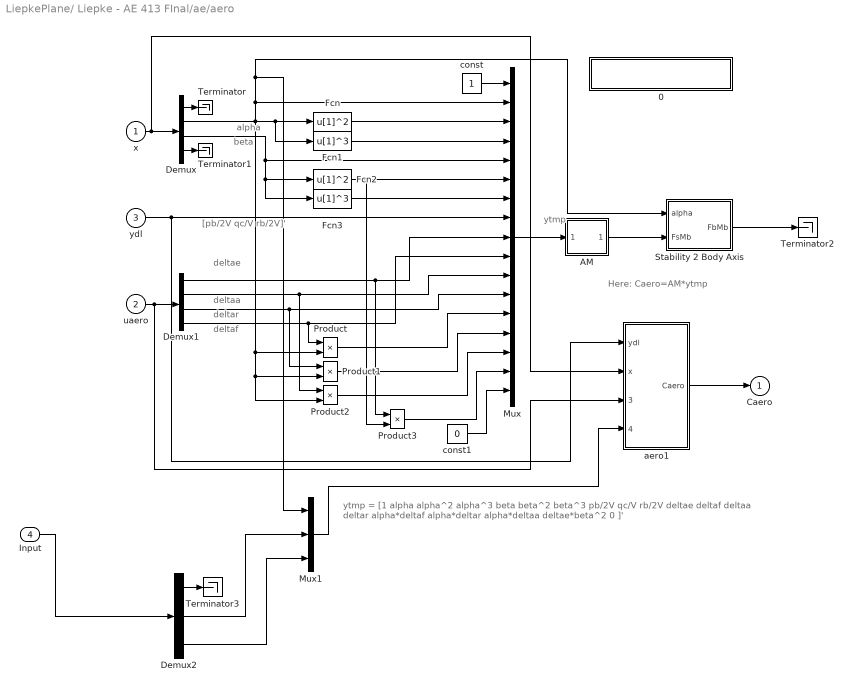
== system LiepkePlane/ Liepke - AE 413 FInal/ae/aero ==
  note: [pb/2V qc/V rb/2V]'
  note: beta
  note: deltaf
  note: ytmp = [1  alpha  alpha^2  alpha^3  beta  beta^2  beta^3  pb/2V  qc/V  rb/2V  deltae
      | deltaf  deltaa  deltar  alpha*deltaf  alpha*deltar  alpha*deltaa  deltae*beta^2  0 ]'
  note: deltaa
  note: deltae
  note: deltar
  note: alpha
  note: ytmp
  note: Here: Caero=AM*ytmp
  x : Inport
  uaero : Inport  Port=2
  ydl : Inport  Port=3
  Input : Inport  Port=4
  0 : Subsystem
      mask Display: disp('AEROMOD\nM.O. Rauw, October 1997')
  "AM " : Subsystem  mask(State Space){M=AM}
      mask prompts: M "Matrix"
      mask Display: disp('Matrix\nGain')
  Demux : Demux  Outputs=[1 1 1 9]
      settings: DisplayOption=none
  Demux1 : Demux
      settings: DisplayOption=none
  Demux2 : Demux  Outputs=3
  Fcn : Fcn  Expr=u[1]^2
  Fcn1 : Fcn  Expr=u[1]^3
  Fcn2 : Fcn  Expr=u[1]^2
  Fcn3 : Fcn  Expr=u[1]^3
  Mux : Mux  Inputs=[1 1 1 1 1 1 1 3 1 1 1 1 1 1 1 1 1]
  Mux1 : Mux  Inputs=3
  Product{,1..3} (4 alike) : Product  InputSameDT=on  RndMeth=Zero  SaturateOnIntegerOverflow=on  OutDataTypeStr=Inherit: Same as first input
  Stability 2 Body Axis : Subsystem
  Terminator{,1..3} (4 alike) : Terminator
  aero1 : Subsystem
      mask Display: disp('Derivatives')
  const : Constant
  const1 : Constant  Value=0
  Caero : Outport  VectorParamsAs1DForOutWhenUnconnected=off
  wires:
  ydl/1 -> aero1/1(ydl), Mux/8
  "AM "/1(Out1) -> Stability 2 Body Axis/2(FsMb)
  Stability 2 Body Axis/1(FbMb) -> Terminator2/1
  Fcn/1 -> Mux/3
  Mux/1 -> "AM "/1(In1)
  Demux/2 -> Fcn/1, Fcn1/1, Product/2, Product1/2, Product2/2, Mux/2, Mux1/1, Stability 2 Body Axis/1(alpha)
  x/1 -> aero1/2(x), Demux/1
  Fcn3/1 -> Mux/7
  Demux1/2 -> Mux/11, Product2/1
  Product2/1 -> Mux/15
  const1/1 -> Mux/17
  Fcn1/1 -> Mux/4
  Demux/1 -> Terminator/1
  aero1/1(Caero) -> Caero/1
  uaero/1 -> aero1/3(Controls), Demux1/1
  Product3/1 -> Mux/16
  Demux1/4 -> Mux/10, Product/1
  Fcn2/1 -> Mux/6, Product3/2
  Demux/3 -> Mux/5, Fcn2/1, Fcn3/1
  Demux1/1 -> Mux/9, Product3/1
  Product1/1 -> Mux/14
  const/1 -> Mux/1
  Demux1/3 -> Mux/12, Product1/1
  Demux/4 -> Terminator1/1
  Product/1 -> Mux/13
  Input/1 -> Demux2/1
  Demux2/2 -> Mux1/2
  Demux2/3 -> Mux1/3
  Mux1/1 -> aero1/4("[alpha,mach,alt]")
  Demux2/1 -> Terminator3/1

== system LiepkePlane/ Liepke - AE 413 FInal/ae/dl ==
  x : Inport
  0 : Subsystem
      mask Display: disp('DIMLESS\nM.O. Rauw, October 1997')
  Mux : Mux  Inputs=3
  pb/2V : Fcn  Expr=0.5 * u[4] * b / u[1]
  qc/2V : Fcn  Expr=0.5* u[5] * cbar / u[1]
  rb/2V : Fcn  Expr=0.5 * u[6] * b / u[1]
  ydl : Outport
  wires:
  pb/2V/1 -> Mux/1
  qc/2V/1 -> Mux/2
  rb/2V/1 -> Mux/3
  Mux/1 -> ydl/1
  x/1 -> qc/2V/1, rb/2V/1, pb/2V/1

== system LiepkePlane/ Liepke - AE 413 FInal/ae/fmdims ==
  yad1 : Inport
  Force / moment derivatives : Inport  Port=2
  0 : Subsystem
      mask Display: disp('FMDIMS\nM.O. Rauw, October 1997')
  Mux : Mux  Inputs=[3 6]
  Mux1 : Mux  Inputs=6
  S : Gain  Gain=S  SaturateOnIntegerOverflow=on  OutDataTypeStr=Inherit: Same as input  ParamDataTypeStr=Inherit: Same as input
  b : Gain  Gain=b  SaturateOnIntegerOverflow=on  OutDataTypeStr=Inherit: Same as input  ParamDataTypeStr=Inherit: Same as input
  "b " : Gain  Gain=b  SaturateOnIntegerOverflow=on  OutDataTypeStr=Inherit: Same as input  ParamDataTypeStr=Inherit: Same as input
  cbar : Gain  Gain=cbar  SaturateOnIntegerOverflow=on  OutDataTypeStr=Inherit: Same as input  ParamDataTypeStr=Inherit: Same as input
  qdyn * S * CX : Fcn  Expr=u[4]*u[3]
  qdyn * S * CY : Fcn  Expr=u[5]*u[3]
  qdyn * S * CZ : Fcn  Expr=u[6]*u[3]
  qdyn * S * Cl : Fcn  Expr=u[7]*u[3]
  qdyn * S * Cm : Fcn  Expr=u[8]*u[3]
  qdyn * S * Cn : Fcn  Expr=u[9]*u[3]
  Forces and moments : Outport
  wires:
  Mux1/1 -> Forces and moments/1
  "b "/1 -> Mux1/6
  cbar/1 -> Mux1/5
  Force / moment derivatives/1 -> S/1
  Mux/1 -> qdyn * S * CZ/1, qdyn * S * CX/1, qdyn * S * CY/1, qdyn * S * Cl/1, qdyn * S * Cm/1, qdyn * S * Cn/1
  qdyn * S * Cl/1 -> b/1
  qdyn * S * Cm/1 -> cbar/1
  qdyn * S * Cn/1 -> "b "/1
  yad1/1 -> Mux/1
  qdyn * S * CX/1 -> Mux1/1
  qdyn * S * CY/1 -> Mux1/2
  S/1 -> Mux/2
  qdyn * S * CZ/1 -> Mux1/3
  b/1 -> Mux1/4

== system LiepkePlane/ Liepke - AE 413 FInal/eqm/0 ==

== system LiepkePlane/ Liepke - AE 413 FInal/eqm/? ==

== system LiepkePlane/ Liepke - AE 413 FInal/eqm/ODE ==
  x : Inport
  Ftot : Inport  Port=2
  Mtot : Inport  Port=3
  yhlp : Inport  Port=4
  ybvel* : Inport  Port=5
  0 : Subsystem
      mask Display: disp('12 Ordinary Differential\nEquations (level 4)\nM.O. Rauw')
  Eulerdot : Subsystem  mask(Eulerdot){}
      mask help:
      | Calculation of d(psi)/dt, d(theta)/dt,
      | and d(phi/dt)
      mask Display: disp('psi dot\ntheta dot\nphi dot')
  Mux : Mux  Inputs=[12 3 3 11]
  Mux1 : Mux  Inputs=[3 3 3 3]
  Vabdot : Subsystem  mask(Vabdot){m=GM1(10)}
      mask prompts: m "Mass of the aircraft [kg]:"
      mask help: Calculation of dV/dt, dalpha/dt, dbeta/dt.
      mask Display: disp('V dot\nalpha dot\nbeta dot')
  pqrdot : Subsystem  mask(pqrdot){}
      mask help: Calculation of dp/dt, dq/dt, and dr/dt
      mask Display: disp('p dot\nq dot\nr dot')
  xyHdot : Subsystem  mask(xyHdot){}
      mask help: Calculation of d(xe)/dt, d(ye)/dt, and dH/dt
      mask Display: disp('xe dot\nye dot\nH dot')
  xdot : Outport
  wires:
  x/1 -> Mux/1
  Mtot/1 -> Mux/3
  Ftot/1 -> Mux/2
  Mux/1 -> pqrdot/1(upqr), Vabdot/1(uVab), Eulerdot/1(ueul), xyHdot/2(uxYH)
  ybvel*/1 -> xyHdot/1(ybvel*)
  yhlp/1 -> Mux/4
  xyHdot/1(yxyH) -> Mux1/4
  Eulerdot/1(yeul) -> Mux1/3
  pqrdot/1(ypqr) -> Mux1/2
  Vabdot/1(yVab) -> Mux1/1
  Mux1/1 -> xdot/1

== system LiepkePlane/ Liepke - AE 413 FInal/eqm/uvw ==
  yhlp : Inport
  x : Inport  Port=2
  0 : Subsystem
      mask Display: disp('UVW\nM.O. Rauw, October 1997')
  Mux : Mux  Inputs=3
  Mux1 : Mux  Inputs=[12 11]
  u : Fcn  Expr=u[1]*u[13]*u[15]
  v : Fcn  Expr=u[1]*u[16]
  w : Fcn  Expr=u[1]*u[14]*u[15]
  ybvel : Outport
  wires:
  Mux1/1 -> v/1, u/1, w/1
  yhlp/1 -> Mux1/2
  x/1 -> Mux1/1
  u/1 -> Mux/1
  v/1 -> Mux/2
  w/1 -> Mux/3
  Mux/1 -> ybvel/1

== system LiepkePlane/ Liepke - AE 413 FInal/eqm/xdotcorr ==
  xdot uncorrected : Inport
  yhlp : Inport  Port=2
  yatm : Inport  Port=3
  0 : Subsystem
      mask Display: disp('XDOTCORR (General)\nM.O. Rauw, October 1997')
  Demux : Demux  Outputs=12
      settings: DisplayOption=none
  Mux1 : Mux  Inputs=12
  Mux2 : Mux  Inputs=[11 1 5]
  beta dot correction : Fcn  Expr=u[12] / (1 - (u[3]*u[13]*b*S*CYbdot)/(4*m))
  xdot corrected : Outport
  wires:
  beta dot correction/1 -> Mux1/3
  yatm/1 -> Mux2/3
  Demux/1 -> Mux1/1
  Demux/2 -> Mux1/2
  Demux/4 -> Mux1/4
  Demux/5 -> Mux1/5
  Demux/6 -> Mux1/6
  Demux/7 -> Mux1/7
  Demux/8 -> Mux1/8
  Demux/9 -> Mux1/9
  Demux/10 -> Mux1/10
  Demux/11 -> Mux1/11
  Demux/12 -> Mux1/12
  Demux/3 -> Mux2/2
  xdot uncorrected/1 -> Demux/1
  Mux1/1 -> xdot corrected/1
  Mux2/1 -> beta dot correction/1
  yhlp/1 -> Mux2/1

== system LiepkePlane/ Liepke - AE 413 FInal/fms/0 ==

== system LiepkePlane/ Liepke - AE 413 FInal/fw/0 ==

== system LiepkePlane/ Liepke - AE 413 FInal/gr/0 ==

== system LiepkePlane/ Liepke - AE 413 FInal/hlp/0 ==

== system LiepkePlane/ Liepke - AE 413 FInal/out/0 ==

== system LiepkePlane/ Liepke - AE 413 FInal/out/accel ==
  Ftot : Inport
  Fgrav : Inport  Port=2
  0 : Subsystem
      mask Display: disp('ACCEL\nM.O. Rauw, October 1997')
  Ax : Fcn  Expr=(u[1]-u[4])/(m*9.80665)
  Ay : Fcn  Expr=(u[2]-u[5])/(m*9.80665)
  Az : Fcn  Expr=(u[3]-u[6])/(m*9.80665)
  Mux : Mux  Inputs=6
  Mux1 : Mux  Inputs=[3 3]
  axk : Fcn  Expr=u[1]/(m*9.80665)
  ayk : Fcn  Expr=u[2]/(m*9.80665)
  azk : Fcn  Expr=u[3]/(m*9.80665)
  yacc : Outport
  wires:
  Ftot/1 -> Mux1/1
  Fgrav/1 -> Mux1/2
  Mux/1 -> yacc/1
  azk/1 -> Mux/6
  Az/1 -> Mux/3
  Ay/1 -> Mux/2
  Ax/1 -> Mux/1
  Mux1/1 -> Az/1, Ax/1, Ay/1, axk/1, azk/1, ayk/1
  axk/1 -> Mux/4
  ayk/1 -> Mux/5

== system LiepkePlane/ Liepke - AE 413 FInal/out/fp ==
  x : Inport
  xdot : Inport  Port=2
  0 : Subsystem
      mask Display: disp('FLPATH\nM.O. Rauw, October 1997')
  Mux : Mux  Inputs=[12 12]
  Mux1 : Mux
  Phi : Fcn  Expr=u[9]*cos(u[8]-alpha0)
  chi : Fcn  Expr=u[3]+u[7]
  fpa : Fcn  Expr=u[13]/9.80665
  gamma : Fcn  Expr=asin(u[24]/u[1])
  yfp : Outport
  wires:
  gamma/1 -> Mux1/1
  Mux/1 -> chi/1, Phi/1, fpa/1, gamma/1
  fpa/1 -> Mux1/2
  chi/1 -> Mux1/3
  Phi/1 -> Mux1/4
  Mux1/1 -> yfp/1
  x/1 -> Mux/1
  xdot/1 -> Mux/2

== system LiepkePlane/ Liepke - AE 413 FInal/out/uvwdot ==
  note: `
  note: cos(alpha)
  note: sin(alpha)
  note: cos(beta)
  note: sin(beta)
  note: V
  x : Inport
  xdot : Inport  Port=2
  yhlp : Inport  Port=3
  0 : Subsystem
      mask Display: disp('UVWDOT\nM.O. Rauw, October 1997')
  DeMux : Demux  Outputs=[1 1 1 1 7]
      settings: DisplayOption=none
  Demux : Demux  Outputs=[1 11]
      settings: DisplayOption=none
  Mux : Mux  Inputs=[1 1 1 1 1 12]
  Mux1 : Mux  Inputs=3
  Terminator : Terminator
  Terminator1 : Terminator
  u dot : Fcn  Expr=u[6]*u[1]*u[3] - u[5]*(u[7]*u[2]*u[3] + u[8]*u[1]*u[4])
  v dot : Fcn  Expr=u[6]*u[4] + u[5]*u[3]*u[8]
  wdot : Fcn  Expr=u[6]*u[2]*u[3] + u[5]*(u[7]*u[1]*u[3] - u[8]*u[2]*u[4])
  yuvw = [udot; vdot; wdot] : Outport
  wires:
  Demux/2 -> Terminator1/1
  DeMux/5 -> Terminator/1
  wdot/1 -> Mux1/3
  v dot/1 -> Mux1/2
  u dot/1 -> Mux1/1
  xdot/1 -> Mux/6
  Mux/1 -> v dot/1, wdot/1, u dot/1
  DeMux/1 -> Mux/1
  DeMux/2 -> Mux/2
  x/1 -> Demux/1
  Mux1/1 -> yuvw = [udot; vdot; wdot]/1
  yhlp/1 -> DeMux/1
  DeMux/3 -> Mux/3
  DeMux/4 -> Mux/4
  Demux/1 -> Mux/5

== system LiepkePlane/ Liepke - AE 413 FInal/ad/ad1/0 ==

== system LiepkePlane/ Liepke - AE 413 FInal/ad/ad2/0 ==

== system LiepkePlane/ Liepke - AE 413 FInal/ad/ad3/0 ==

== system LiepkePlane/ Liepke - AE 413 FInal/ad/atm/0 ==

== system LiepkePlane/ Liepke - AE 413 FInal/ae/aero/0 ==

== system LiepkePlane/ Liepke - AE 413 FInal/ae/aero/AM  ==
  In1 : Inport
  Matrix Gain : StateSpace  A=[]  B=[]  C=[]  D=M  InitialCondition=0
  Out1 : Outport  VectorParamsAs1DForOutWhenUnconnected=off
  wires:
  In1/1 -> Matrix Gain/1
  Matrix Gain/1 -> Out1/1
